simulink model "gm_ZynqBF_2tx_fpga"  (R2018b)
settings: Solver=FixedStepDiscrete  StartTime=0.0  StopTime=10.0  FixedStep=(1/420e3)/128  RelTol=1e-3
undefined symbols (not defined in the file or in its folder): a, b, c
libraries: hdlsllib x873, simulink x349
(part 28 of 40)

== system gm_ZynqBF_2tx_fpga/channel_estimator/peakdetect_ch2/correlator2/correlator_q_instance59 ==
  rx : Inport  OutDataTypeStr=fixdt(1, 16, 15)  PortDimensions=1  SampleTime=1.86011904761905e-08
  gs : Inport  Port=2  OutDataTypeStr=fixdt(1, 16, 15)  PortDimensions=1  SampleTime=1.86011904761905e-08
  start : Inport  Port=3  OutDataTypeStr=boolean  PortDimensions=1  SampleTime=1.86011904761905e-08
  vin : Inport  Port=4  OutDataTypeStr=boolean  PortDimensions=1  SampleTime=1.86011904761905e-08
  Compare To Constant1 : simulink/Logic and Bit Operations/Compare To Constant  relop===  const=fi(0,0,7,0,'hex','3f')  OutDataTypeStr=boolean
  Constant : Constant  Value=0  OutDataTypeStr=fixdt(1, 32, 16)  SampleTime=-1
  Constant1 : Constant  Value=0  OutDataTypeStr=fixdt(1, 16, 15)  SampleTime=-1
  Delay1 : Delay  DelayLength=double(1)  InitialCondition=0  InputProcessing=Inherited  SampleTime=1.86011904761905e-08
  HDL Counter : hdlsllib/Sources/HDL Counter  CountType=Free running  CountInit=double(0)  CountStep=double(1)  CountMax=25  CountFromType=Initial value  CountFrom=double(0)  CountResetPort=on  CountLoadPort=off  CountEnbPort=on  CountDirPort=off  CountDataType=Unsigned  CountWordLen=7  CountFracLen=0  CountSampTime=1.86011904761905e-08
      settings: SourceProductBaseCode=HD
  Multiply-Add : hdlsllib/HDL Operations/Multiply-Add  Function=c+(a.*b)  datatype=fixdt(1, 32, 16)  DoSatur=off  FMA=off
      settings: SourceProductName=HDL Coder  SourceProductBaseCode=HD
  Switch : Switch  Criteria=u2 ~= 0  Threshold=double(0)  OutDataTypeStr=fixdt(1, 32, 16)  SampleTime=1.86011904761905e-08
  Switch1 : Switch  Criteria=u2 ~= 0  Threshold=double(0)  OutDataTypeStr=fixdt(1, 16, 15)  SampleTime=1.86011904761905e-08
  Switch2 : Switch  Criteria=u2 ~= 0  Threshold=double(0)  OutDataTypeStr=fixdt(1, 16, 15)  SampleTime=1.86011904761905e-08
  dout : Outport
  vout : Outport  Port=2
  wires:
  Switch/1 -> Multiply-Add/3
  Delay1/1 -> Switch/3
  vin/1 -> HDL Counter/2, Switch2/2, Switch1/2
  start/1 -> Switch/2, HDL Counter/1
  gs/1 -> Switch2/1
  rx/1 -> Switch1/1
  Compare To Constant1/1 -> vout/1
  Constant/1 -> Switch/1
  Constant1/1 -> Switch2/3, Switch1/3
  HDL Counter/1 -> Compare To Constant1/1
  Multiply-Add/1 -> Delay1/1, dout/1
  Switch1/1 -> Multiply-Add/1
  Switch2/1 -> Multiply-Add/2

== system gm_ZynqBF_2tx_fpga/channel_estimator/peakdetect_ch2/correlator2/correlator_q_instance6 ==
  rx : Inport  OutDataTypeStr=fixdt(1, 16, 15)  PortDimensions=1  SampleTime=1.86011904761905e-08
  gs : Inport  Port=2  OutDataTypeStr=fixdt(1, 16, 15)  PortDimensions=1  SampleTime=1.86011904761905e-08
  start : Inport  Port=3  OutDataTypeStr=boolean  PortDimensions=1  SampleTime=1.86011904761905e-08
  vin : Inport  Port=4  OutDataTypeStr=boolean  PortDimensions=1  SampleTime=1.86011904761905e-08
  Compare To Constant1 : simulink/Logic and Bit Operations/Compare To Constant  relop===  const=fi(0,0,7,0,'hex','3f')  OutDataTypeStr=boolean
  Constant : Constant  Value=0  OutDataTypeStr=fixdt(1, 32, 16)  SampleTime=-1
  Constant1 : Constant  Value=0  OutDataTypeStr=fixdt(1, 16, 15)  SampleTime=-1
  Delay1 : Delay  DelayLength=double(1)  InitialCondition=0  InputProcessing=Inherited  SampleTime=1.86011904761905e-08
  HDL Counter : hdlsllib/Sources/HDL Counter  CountType=Free running  CountInit=double(0)  CountStep=double(1)  CountMax=25  CountFromType=Initial value  CountFrom=double(0)  CountResetPort=on  CountLoadPort=off  CountEnbPort=on  CountDirPort=off  CountDataType=Unsigned  CountWordLen=7  CountFracLen=0  CountSampTime=1.86011904761905e-08
      settings: SourceProductBaseCode=HD
  Multiply-Add : hdlsllib/HDL Operations/Multiply-Add  Function=c+(a.*b)  datatype=fixdt(1, 32, 16)  DoSatur=off  FMA=off
      settings: SourceProductName=HDL Coder  SourceProductBaseCode=HD
  Switch : Switch  Criteria=u2 ~= 0  Threshold=double(0)  OutDataTypeStr=fixdt(1, 32, 16)  SampleTime=1.86011904761905e-08
  Switch1 : Switch  Criteria=u2 ~= 0  Threshold=double(0)  OutDataTypeStr=fixdt(1, 16, 15)  SampleTime=1.86011904761905e-08
  Switch2 : Switch  Criteria=u2 ~= 0  Threshold=double(0)  OutDataTypeStr=fixdt(1, 16, 15)  SampleTime=1.86011904761905e-08
  dout : Outport
  vout : Outport  Port=2
  wires:
  Switch/1 -> Multiply-Add/3
  Delay1/1 -> Switch/3
  vin/1 -> HDL Counter/2, Switch2/2, Switch1/2
  start/1 -> Switch/2, HDL Counter/1
  gs/1 -> Switch2/1
  rx/1 -> Switch1/1
  Compare To Constant1/1 -> vout/1
  Constant/1 -> Switch/1
  Constant1/1 -> Switch2/3, Switch1/3
  HDL Counter/1 -> Compare To Constant1/1
  Multiply-Add/1 -> Delay1/1, dout/1
  Switch1/1 -> Multiply-Add/1
  Switch2/1 -> Multiply-Add/2

== system gm_ZynqBF_2tx_fpga/channel_estimator/peakdetect_ch2/correlator2/correlator_q_instance60 ==
  rx : Inport  OutDataTypeStr=fixdt(1, 16, 15)  PortDimensions=1  SampleTime=1.86011904761905e-08
  gs : Inport  Port=2  OutDataTypeStr=fixdt(1, 16, 15)  PortDimensions=1  SampleTime=1.86011904761905e-08
  start : Inport  Port=3  OutDataTypeStr=boolean  PortDimensions=1  SampleTime=1.86011904761905e-08
  vin : Inport  Port=4  OutDataTypeStr=boolean  PortDimensions=1  SampleTime=1.86011904761905e-08
  Compare To Constant1 : simulink/Logic and Bit Operations/Compare To Constant  relop===  const=fi(0,0,7,0,'hex','3f')  OutDataTypeStr=boolean
  Constant : Constant  Value=0  OutDataTypeStr=fixdt(1, 32, 16)  SampleTime=-1
  Constant1 : Constant  Value=0  OutDataTypeStr=fixdt(1, 16, 15)  SampleTime=-1
  Delay1 : Delay  DelayLength=double(1)  InitialCondition=0  InputProcessing=Inherited  SampleTime=1.86011904761905e-08
  HDL Counter : hdlsllib/Sources/HDL Counter  CountType=Free running  CountInit=double(0)  CountStep=double(1)  CountMax=25  CountFromType=Initial value  CountFrom=double(0)  CountResetPort=on  CountLoadPort=off  CountEnbPort=on  CountDirPort=off  CountDataType=Unsigned  CountWordLen=7  CountFracLen=0  CountSampTime=1.86011904761905e-08
      settings: SourceProductBaseCode=HD
  Multiply-Add : hdlsllib/HDL Operations/Multiply-Add  Function=c+(a.*b)  datatype=fixdt(1, 32, 16)  DoSatur=off  FMA=off
      settings: SourceProductName=HDL Coder  SourceProductBaseCode=HD
  Switch : Switch  Criteria=u2 ~= 0  Threshold=double(0)  OutDataTypeStr=fixdt(1, 32, 16)  SampleTime=1.86011904761905e-08
  Switch1 : Switch  Criteria=u2 ~= 0  Threshold=double(0)  OutDataTypeStr=fixdt(1, 16, 15)  SampleTime=1.86011904761905e-08
  Switch2 : Switch  Criteria=u2 ~= 0  Threshold=double(0)  OutDataTypeStr=fixdt(1, 16, 15)  SampleTime=1.86011904761905e-08
  dout : Outport
  vout : Outport  Port=2
  wires:
  Switch/1 -> Multiply-Add/3
  Delay1/1 -> Switch/3
  vin/1 -> HDL Counter/2, Switch2/2, Switch1/2
  start/1 -> Switch/2, HDL Counter/1
  gs/1 -> Switch2/1
  rx/1 -> Switch1/1
  Compare To Constant1/1 -> vout/1
  Constant/1 -> Switch/1
  Constant1/1 -> Switch2/3, Switch1/3
  HDL Counter/1 -> Compare To Constant1/1
  Multiply-Add/1 -> Delay1/1, dout/1
  Switch1/1 -> Multiply-Add/1
  Switch2/1 -> Multiply-Add/2

== system gm_ZynqBF_2tx_fpga/channel_estimator/peakdetect_ch2/correlator2/correlator_q_instance61 ==
  rx : Inport  OutDataTypeStr=fixdt(1, 16, 15)  PortDimensions=1  SampleTime=1.86011904761905e-08
  gs : Inport  Port=2  OutDataTypeStr=fixdt(1, 16, 15)  PortDimensions=1  SampleTime=1.86011904761905e-08
  start : Inport  Port=3  OutDataTypeStr=boolean  PortDimensions=1  SampleTime=1.86011904761905e-08
  vin : Inport  Port=4  OutDataTypeStr=boolean  PortDimensions=1  SampleTime=1.86011904761905e-08
  Compare To Constant1 : simulink/Logic and Bit Operations/Compare To Constant  relop===  const=fi(0,0,7,0,'hex','3f')  OutDataTypeStr=boolean
  Constant : Constant  Value=0  OutDataTypeStr=fixdt(1, 32, 16)  SampleTime=-1
  Constant1 : Constant  Value=0  OutDataTypeStr=fixdt(1, 16, 15)  SampleTime=-1
  Delay1 : Delay  DelayLength=double(1)  InitialCondition=0  InputProcessing=Inherited  SampleTime=1.86011904761905e-08
  HDL Counter : hdlsllib/Sources/HDL Counter  CountType=Free running  CountInit=double(0)  CountStep=double(1)  CountMax=25  CountFromType=Initial value  CountFrom=double(0)  CountResetPort=on  CountLoadPort=off  CountEnbPort=on  CountDirPort=off  CountDataType=Unsigned  CountWordLen=7  CountFracLen=0  CountSampTime=1.86011904761905e-08
      settings: SourceProductBaseCode=HD
  Multiply-Add : hdlsllib/HDL Operations/Multiply-Add  Function=c+(a.*b)  datatype=fixdt(1, 32, 16)  DoSatur=off  FMA=off
      settings: SourceProductName=HDL Coder  SourceProductBaseCode=HD
  Switch : Switch  Criteria=u2 ~= 0  Threshold=double(0)  OutDataTypeStr=fixdt(1, 32, 16)  SampleTime=1.86011904761905e-08
  Switch1 : Switch  Criteria=u2 ~= 0  Threshold=double(0)  OutDataTypeStr=fixdt(1, 16, 15)  SampleTime=1.86011904761905e-08
  Switch2 : Switch  Criteria=u2 ~= 0  Threshold=double(0)  OutDataTypeStr=fixdt(1, 16, 15)  SampleTime=1.86011904761905e-08
  dout : Outport
  vout : Outport  Port=2
  wires:
  Switch/1 -> Multiply-Add/3
  Delay1/1 -> Switch/3
  vin/1 -> HDL Counter/2, Switch2/2, Switch1/2
  start/1 -> Switch/2, HDL Counter/1
  gs/1 -> Switch2/1
  rx/1 -> Switch1/1
  Compare To Constant1/1 -> vout/1
  Constant/1 -> Switch/1
  Constant1/1 -> Switch2/3, Switch1/3
  HDL Counter/1 -> Compare To Constant1/1
  Multiply-Add/1 -> Delay1/1, dout/1
  Switch1/1 -> Multiply-Add/1
  Switch2/1 -> Multiply-Add/2

== system gm_ZynqBF_2tx_fpga/channel_estimator/peakdetect_ch2/correlator2/correlator_q_instance62 ==
  rx : Inport  OutDataTypeStr=fixdt(1, 16, 15)  PortDimensions=1  SampleTime=1.86011904761905e-08
  gs : Inport  Port=2  OutDataTypeStr=fixdt(1, 16, 15)  PortDimensions=1  SampleTime=1.86011904761905e-08
  start : Inport  Port=3  OutDataTypeStr=boolean  PortDimensions=1  SampleTime=1.86011904761905e-08
  vin : Inport  Port=4  OutDataTypeStr=boolean  PortDimensions=1  SampleTime=1.86011904761905e-08
  Compare To Constant1 : simulink/Logic and Bit Operations/Compare To Constant  relop===  const=fi(0,0,7,0,'hex','3f')  OutDataTypeStr=boolean
  Constant : Constant  Value=0  OutDataTypeStr=fixdt(1, 32, 16)  SampleTime=-1
  Constant1 : Constant  Value=0  OutDataTypeStr=fixdt(1, 16, 15)  SampleTime=-1
  Delay1 : Delay  DelayLength=double(1)  InitialCondition=0  InputProcessing=Inherited  SampleTime=1.86011904761905e-08
  HDL Counter : hdlsllib/Sources/HDL Counter  CountType=Free running  CountInit=double(0)  CountStep=double(1)  CountMax=25  CountFromType=Initial value  CountFrom=double(0)  CountResetPort=on  CountLoadPort=off  CountEnbPort=on  CountDirPort=off  CountDataType=Unsigned  CountWordLen=7  CountFracLen=0  CountSampTime=1.86011904761905e-08
      settings: SourceProductBaseCode=HD
  Multiply-Add : hdlsllib/HDL Operations/Multiply-Add  Function=c+(a.*b)  datatype=fixdt(1, 32, 16)  DoSatur=off  FMA=off
      settings: SourceProductName=HDL Coder  SourceProductBaseCode=HD
  Switch : Switch  Criteria=u2 ~= 0  Threshold=double(0)  OutDataTypeStr=fixdt(1, 32, 16)  SampleTime=1.86011904761905e-08
  Switch1 : Switch  Criteria=u2 ~= 0  Threshold=double(0)  OutDataTypeStr=fixdt(1, 16, 15)  SampleTime=1.86011904761905e-08
  Switch2 : Switch  Criteria=u2 ~= 0  Threshold=double(0)  OutDataTypeStr=fixdt(1, 16, 15)  SampleTime=1.86011904761905e-08
  dout : Outport
  vout : Outport  Port=2
  wires:
  Switch/1 -> Multiply-Add/3
  Delay1/1 -> Switch/3
  vin/1 -> HDL Counter/2, Switch2/2, Switch1/2
  start/1 -> Switch/2, HDL Counter/1
  gs/1 -> Switch2/1
  rx/1 -> Switch1/1
  Compare To Constant1/1 -> vout/1
  Constant/1 -> Switch/1
  Constant1/1 -> Switch2/3, Switch1/3
  HDL Counter/1 -> Compare To Constant1/1
  Multiply-Add/1 -> Delay1/1, dout/1
  Switch1/1 -> Multiply-Add/1
  Switch2/1 -> Multiply-Add/2

== system gm_ZynqBF_2tx_fpga/channel_estimator/peakdetect_ch2/correlator2/correlator_q_instance63 ==
  rx : Inport  OutDataTypeStr=fixdt(1, 16, 15)  PortDimensions=1  SampleTime=1.86011904761905e-08
  gs : Inport  Port=2  OutDataTypeStr=fixdt(1, 16, 15)  PortDimensions=1  SampleTime=1.86011904761905e-08
  start : Inport  Port=3  OutDataTypeStr=boolean  PortDimensions=1  SampleTime=1.86011904761905e-08
  vin : Inport  Port=4  OutDataTypeStr=boolean  PortDimensions=1  SampleTime=1.86011904761905e-08
  Compare To Constant1 : simulink/Logic and Bit Operations/Compare To Constant  relop===  const=fi(0,0,7,0,'hex','3f')  OutDataTypeStr=boolean
  Constant : Constant  Value=0  OutDataTypeStr=fixdt(1, 32, 16)  SampleTime=-1
  Constant1 : Constant  Value=0  OutDataTypeStr=fixdt(1, 16, 15)  SampleTime=-1
  Delay1 : Delay  DelayLength=double(1)  InitialCondition=0  InputProcessing=Inherited  SampleTime=1.86011904761905e-08
  HDL Counter : hdlsllib/Sources/HDL Counter  CountType=Free running  CountInit=double(0)  CountStep=double(1)  CountMax=25  CountFromType=Initial value  CountFrom=double(0)  CountResetPort=on  CountLoadPort=off  CountEnbPort=on  CountDirPort=off  CountDataType=Unsigned  CountWordLen=7  CountFracLen=0  CountSampTime=1.86011904761905e-08
      settings: SourceProductBaseCode=HD
  Multiply-Add : hdlsllib/HDL Operations/Multiply-Add  Function=c+(a.*b)  datatype=fixdt(1, 32, 16)  DoSatur=off  FMA=off
      settings: SourceProductName=HDL Coder  SourceProductBaseCode=HD
  Switch : Switch  Criteria=u2 ~= 0  Threshold=double(0)  OutDataTypeStr=fixdt(1, 32, 16)  SampleTime=1.86011904761905e-08
  Switch1 : Switch  Criteria=u2 ~= 0  Threshold=double(0)  OutDataTypeStr=fixdt(1, 16, 15)  SampleTime=1.86011904761905e-08
  Switch2 : Switch  Criteria=u2 ~= 0  Threshold=double(0)  OutDataTypeStr=fixdt(1, 16, 15)  SampleTime=1.86011904761905e-08
  dout : Outport
  vout : Outport  Port=2
  wires:
  Switch/1 -> Multiply-Add/3
  Delay1/1 -> Switch/3
  vin/1 -> HDL Counter/2, Switch2/2, Switch1/2
  start/1 -> Switch/2, HDL Counter/1
  gs/1 -> Switch2/1
  rx/1 -> Switch1/1
  Compare To Constant1/1 -> vout/1
  Constant/1 -> Switch/1
  Constant1/1 -> Switch2/3, Switch1/3
  HDL Counter/1 -> Compare To Constant1/1
  Multiply-Add/1 -> Delay1/1, dout/1
  Switch1/1 -> Multiply-Add/1
  Switch2/1 -> Multiply-Add/2

== system gm_ZynqBF_2tx_fpga/channel_estimator/peakdetect_ch2/correlator2/correlator_q_instance64 ==
  rx : Inport  OutDataTypeStr=fixdt(1, 16, 15)  PortDimensions=1  SampleTime=1.86011904761905e-08
  gs : Inport  Port=2  OutDataTypeStr=fixdt(1, 16, 15)  PortDimensions=1  SampleTime=1.86011904761905e-08
  start : Inport  Port=3  OutDataTypeStr=boolean  PortDimensions=1  SampleTime=1.86011904761905e-08
  vin : Inport  Port=4  OutDataTypeStr=boolean  PortDimensions=1  SampleTime=1.86011904761905e-08
  Compare To Constant1 : simulink/Logic and Bit Operations/Compare To Constant  relop===  const=fi(0,0,7,0,'hex','3f')  OutDataTypeStr=boolean
  Constant : Constant  Value=0  OutDataTypeStr=fixdt(1, 32, 16)  SampleTime=-1
  Constant1 : Constant  Value=0  OutDataTypeStr=fixdt(1, 16, 15)  SampleTime=-1
  Delay1 : Delay  DelayLength=double(1)  InitialCondition=0  InputProcessing=Inherited  SampleTime=1.86011904761905e-08
  HDL Counter : hdlsllib/Sources/HDL Counter  CountType=Free running  CountInit=double(0)  CountStep=double(1)  CountMax=25  CountFromType=Initial value  CountFrom=double(0)  CountResetPort=on  CountLoadPort=off  CountEnbPort=on  CountDirPort=off  CountDataType=Unsigned  CountWordLen=7  CountFracLen=0  CountSampTime=1.86011904761905e-08
      settings: SourceProductBaseCode=HD
  Multiply-Add : hdlsllib/HDL Operations/Multiply-Add  Function=c+(a.*b)  datatype=fixdt(1, 32, 16)  DoSatur=off  FMA=off
      settings: SourceProductName=HDL Coder  SourceProductBaseCode=HD
  Switch : Switch  Criteria=u2 ~= 0  Threshold=double(0)  OutDataTypeStr=fixdt(1, 32, 16)  SampleTime=1.86011904761905e-08
  Switch1 : Switch  Criteria=u2 ~= 0  Threshold=double(0)  OutDataTypeStr=fixdt(1, 16, 15)  SampleTime=1.86011904761905e-08
  Switch2 : Switch  Criteria=u2 ~= 0  Threshold=double(0)  OutDataTypeStr=fixdt(1, 16, 15)  SampleTime=1.86011904761905e-08
  dout : Outport
  vout : Outport  Port=2
  wires:
  Switch/1 -> Multiply-Add/3
  Delay1/1 -> Switch/3
  vin/1 -> HDL Counter/2, Switch2/2, Switch1/2
  start/1 -> Switch/2, HDL Counter/1
  gs/1 -> Switch2/1
  rx/1 -> Switch1/1
  Compare To Constant1/1 -> vout/1
  Constant/1 -> Switch/1
  Constant1/1 -> Switch2/3, Switch1/3
  HDL Counter/1 -> Compare To Constant1/1
  Multiply-Add/1 -> Delay1/1, dout/1
  Switch1/1 -> Multiply-Add/1
  Switch2/1 -> Multiply-Add/2

== system gm_ZynqBF_2tx_fpga/channel_estimator/peakdetect_ch2/correlator2/correlator_q_instance7 ==
  rx : Inport  OutDataTypeStr=fixdt(1, 16, 15)  PortDimensions=1  SampleTime=1.86011904761905e-08
  gs : Inport  Port=2  OutDataTypeStr=fixdt(1, 16, 15)  PortDimensions=1  SampleTime=1.86011904761905e-08
  start : Inport  Port=3  OutDataTypeStr=boolean  PortDimensions=1  SampleTime=1.86011904761905e-08
  vin : Inport  Port=4  OutDataTypeStr=boolean  PortDimensions=1  SampleTime=1.86011904761905e-08
  Compare To Constant1 : simulink/Logic and Bit Operations/Compare To Constant  relop===  const=fi(0,0,7,0,'hex','3f')  OutDataTypeStr=boolean
  Constant : Constant  Value=0  OutDataTypeStr=fixdt(1, 32, 16)  SampleTime=-1
  Constant1 : Constant  Value=0  OutDataTypeStr=fixdt(1, 16, 15)  SampleTime=-1
  Delay1 : Delay  DelayLength=double(1)  InitialCondition=0  InputProcessing=Inherited  SampleTime=1.86011904761905e-08
  HDL Counter : hdlsllib/Sources/HDL Counter  CountType=Free running  CountInit=double(0)  CountStep=double(1)  CountMax=25  CountFromType=Initial value  CountFrom=double(0)  CountResetPort=on  CountLoadPort=off  CountEnbPort=on  CountDirPort=off  CountDataType=Unsigned  CountWordLen=7  CountFracLen=0  CountSampTime=1.86011904761905e-08
      settings: SourceProductBaseCode=HD
  Multiply-Add : hdlsllib/HDL Operations/Multiply-Add  Function=c+(a.*b)  datatype=fixdt(1, 32, 16)  DoSatur=off  FMA=off
      settings: SourceProductName=HDL Coder  SourceProductBaseCode=HD
  Switch : Switch  Criteria=u2 ~= 0  Threshold=double(0)  OutDataTypeStr=fixdt(1, 32, 16)  SampleTime=1.86011904761905e-08
  Switch1 : Switch  Criteria=u2 ~= 0  Threshold=double(0)  OutDataTypeStr=fixdt(1, 16, 15)  SampleTime=1.86011904761905e-08
  Switch2 : Switch  Criteria=u2 ~= 0  Threshold=double(0)  OutDataTypeStr=fixdt(1, 16, 15)  SampleTime=1.86011904761905e-08
  dout : Outport
  vout : Outport  Port=2
  wires:
  Switch/1 -> Multiply-Add/3
  Delay1/1 -> Switch/3
  vin/1 -> HDL Counter/2, Switch2/2, Switch1/2
  start/1 -> Switch/2, HDL Counter/1
  gs/1 -> Switch2/1
  rx/1 -> Switch1/1
  Compare To Constant1/1 -> vout/1
  Constant/1 -> Switch/1
  Constant1/1 -> Switch2/3, Switch1/3
  HDL Counter/1 -> Compare To Constant1/1
  Multiply-Add/1 -> Delay1/1, dout/1
  Switch1/1 -> Multiply-Add/1
  Switch2/1 -> Multiply-Add/2

== system gm_ZynqBF_2tx_fpga/channel_estimator/peakdetect_ch2/correlator2/correlator_q_instance8 ==
  rx : Inport  OutDataTypeStr=fixdt(1, 16, 15)  PortDimensions=1  SampleTime=1.86011904761905e-08
  gs : Inport  Port=2  OutDataTypeStr=fixdt(1, 16, 15)  PortDimensions=1  SampleTime=1.86011904761905e-08
  start : Inport  Port=3  OutDataTypeStr=boolean  PortDimensions=1  SampleTime=1.86011904761905e-08
  vin : Inport  Port=4  OutDataTypeStr=boolean  PortDimensions=1  SampleTime=1.86011904761905e-08
  Compare To Constant1 : simulink/Logic and Bit Operations/Compare To Constant  relop===  const=fi(0,0,7,0,'hex','3f')  OutDataTypeStr=boolean
  Constant : Constant  Value=0  OutDataTypeStr=fixdt(1, 32, 16)  SampleTime=-1
  Constant1 : Constant  Value=0  OutDataTypeStr=fixdt(1, 16, 15)  SampleTime=-1
  Delay1 : Delay  DelayLength=double(1)  InitialCondition=0  InputProcessing=Inherited  SampleTime=1.86011904761905e-08
  HDL Counter : hdlsllib/Sources/HDL Counter  CountType=Free running  CountInit=double(0)  CountStep=double(1)  CountMax=25  CountFromType=Initial value  CountFrom=double(0)  CountResetPort=on  CountLoadPort=off  CountEnbPort=on  CountDirPort=off  CountDataType=Unsigned  CountWordLen=7  CountFracLen=0  CountSampTime=1.86011904761905e-08
      settings: SourceProductBaseCode=HD
  Multiply-Add : hdlsllib/HDL Operations/Multiply-Add  Function=c+(a.*b)  datatype=fixdt(1, 32, 16)  DoSatur=off  FMA=off
      settings: SourceProductName=HDL Coder  SourceProductBaseCode=HD
  Switch : Switch  Criteria=u2 ~= 0  Threshold=double(0)  OutDataTypeStr=fixdt(1, 32, 16)  SampleTime=1.86011904761905e-08
  Switch1 : Switch  Criteria=u2 ~= 0  Threshold=double(0)  OutDataTypeStr=fixdt(1, 16, 15)  SampleTime=1.86011904761905e-08
  Switch2 : Switch  Criteria=u2 ~= 0  Threshold=double(0)  OutDataTypeStr=fixdt(1, 16, 15)  SampleTime=1.86011904761905e-08
  dout : Outport
  vout : Outport  Port=2
  wires:
  Switch/1 -> Multiply-Add/3
  Delay1/1 -> Switch/3
  vin/1 -> HDL Counter/2, Switch2/2, Switch1/2
  start/1 -> Switch/2, HDL Counter/1
  gs/1 -> Switch2/1
  rx/1 -> Switch1/1
  Compare To Constant1/1 -> vout/1
  Constant/1 -> Switch/1
  Constant1/1 -> Switch2/3, Switch1/3
  HDL Counter/1 -> Compare To Constant1/1
  Multiply-Add/1 -> Delay1/1, dout/1
  Switch1/1 -> Multiply-Add/1
  Switch2/1 -> Multiply-Add/2

== system gm_ZynqBF_2tx_fpga/channel_estimator/peakdetect_ch2/correlator2/correlator_q_instance9 ==
  rx : Inport  OutDataTypeStr=fixdt(1, 16, 15)  PortDimensions=1  SampleTime=1.86011904761905e-08
  gs : Inport  Port=2  OutDataTypeStr=fixdt(1, 16, 15)  PortDimensions=1  SampleTime=1.86011904761905e-08
  start : Inport  Port=3  OutDataTypeStr=boolean  PortDimensions=1  SampleTime=1.86011904761905e-08
  vin : Inport  Port=4  OutDataTypeStr=boolean  PortDimensions=1  SampleTime=1.86011904761905e-08
  Compare To Constant1 : simulink/Logic and Bit Operations/Compare To Constant  relop===  const=fi(0,0,7,0,'hex','3f')  OutDataTypeStr=boolean
  Constant : Constant  Value=0  OutDataTypeStr=fixdt(1, 32, 16)  SampleTime=-1
  Constant1 : Constant  Value=0  OutDataTypeStr=fixdt(1, 16, 15)  SampleTime=-1
  Delay1 : Delay  DelayLength=double(1)  InitialCondition=0  InputProcessing=Inherited  SampleTime=1.86011904761905e-08
  HDL Counter : hdlsllib/Sources/HDL Counter  CountType=Free running  CountInit=double(0)  CountStep=double(1)  CountMax=25  CountFromType=Initial value  CountFrom=double(0)  CountResetPort=on  CountLoadPort=off  CountEnbPort=on  CountDirPort=off  CountDataType=Unsigned  CountWordLen=7  CountFracLen=0  CountSampTime=1.86011904761905e-08
      settings: SourceProductBaseCode=HD
  Multiply-Add : hdlsllib/HDL Operations/Multiply-Add  Function=c+(a.*b)  datatype=fixdt(1, 32, 16)  DoSatur=off  FMA=off
      settings: SourceProductName=HDL Coder  SourceProductBaseCode=HD
  Switch : Switch  Criteria=u2 ~= 0  Threshold=double(0)  OutDataTypeStr=fixdt(1, 32, 16)  SampleTime=1.86011904761905e-08
  Switch1 : Switch  Criteria=u2 ~= 0  Threshold=double(0)  OutDataTypeStr=fixdt(1, 16, 15)  SampleTime=1.86011904761905e-08
  Switch2 : Switch  Criteria=u2 ~= 0  Threshold=double(0)  OutDataTypeStr=fixdt(1, 16, 15)  SampleTime=1.86011904761905e-08
  dout : Outport
  vout : Outport  Port=2
  wires:
  Switch/1 -> Multiply-Add/3
  Delay1/1 -> Switch/3
  vin/1 -> HDL Counter/2, Switch2/2, Switch1/2
  start/1 -> Switch/2, HDL Counter/1
  gs/1 -> Switch2/1
  rx/1 -> Switch1/1
  Compare To Constant1/1 -> vout/1
  Constant/1 -> Switch/1
  Constant1/1 -> Switch2/3, Switch1/3
  HDL Counter/1 -> Compare To Constant1/1
  Multiply-Add/1 -> Delay1/1, dout/1
  Switch1/1 -> Multiply-Add/1
  Switch2/1 -> Multiply-Add/2

== system gm_ZynqBF_2tx_fpga/channel_estimator/peakdetect_ch2/correlator2/data_in ==
  rst : Inport  OutDataTypeStr=boolean  PortDimensions=1  SampleTime=1.86011904761905e-08
  valid : Inport  Port=2  OutDataTypeStr=boolean  PortDimensions=1  SampleTime=1.86011904761905e-08
  Bit Rotate : hdlsllib/Logic and Bit Operations/Bit Rotate  mode=Rotate Left  N=double(1)
      settings: SourceProductName=HDL Coder  SourceProductBaseCode=HD
  Compare To Constant : simulink/Logic and Bit Operations/Compare To Constant  relop===  const=fi(0,0,6,0,'hex','3f')  OutDataTypeStr=boolean
  Constant1 : Constant  Value=0  OutDataTypeStr=fixdt(0, 64, 0)  SampleTime=-1
  Delay{,1..4,6} (6 alike) : Delay  DelayLength=double(1)  InitialCondition=0  InputProcessing=Inherited  SampleTime=1.86011904761905e-08
  Delay1_Initial_Val : Constant  Value=9223372036854775808  OutDataTypeStr=fixdt(0, 64, 0)  SampleTime=-1
  Delay1_ctrl_const : Constant  OutDataTypeStr=boolean  SampleTime=1.86011904761905e-08
  Delay1_ctrl_delay : Delay  DelayLength=double(1)  InitialCondition=0  InputProcessing=Inherited  SampleTime=1.86011904761905e-08
  Delay1_switch : Switch  Criteria=u2 ~= 0  Threshold=double(0)  OutDataTypeStr=fixdt(0, 64, 0)  SampleTime=1.86011904761905e-08
  Delay5 : Delay  DelayLength=double(3)  InitialCondition=0  InputProcessing=Inherited  SampleTime=1.86011904761905e-08
  Logical Operator : Logic  AllPortsSameDT=off  OutDataTypeStr=boolean  SampleTime=1.86011904761905e-08
  Switch1 : Switch  Criteria=u2 ~= 0  Threshold=double(0)  OutDataTypeStr=fixdt(0, 64, 0)  SampleTime=1.86011904761905e-08
  Switch2 : Switch  Criteria=u2 ~= 0  Threshold=double(0)  OutDataTypeStr=fixdt(0, 64, 0)  SampleTime=1.86011904761905e-08
  addr_counter : hdlsllib/Sources/HDL Counter  CountType=Count limited  CountInit=double(63)  CountStep=double(1)  CountMax=double(511)  CountFromType=Initial value  CountFrom=double(63)  CountResetPort=on  CountLoadPort=off  CountEnbPort=on  CountDirPort=off  CountDataType=Unsigned  CountWordLen=9  CountFracLen=0  CountSampTime=1.86011904761905e-08
      settings: SourceProductBaseCode=HD
  ram_counter : hdlsllib/Sources/HDL Counter  CountType=Free running  CountInit=double(63)  CountStep=double(1)  CountMax=25  CountFromType=Initial value  CountFrom=double(63)  CountResetPort=on  CountLoadPort=off  CountEnbPort=on  CountDirPort=off  CountDataType=Unsigned  CountWordLen=6  CountFracLen=0  CountSampTime=1.86011904761905e-08
      settings: SourceProductBaseCode=HD
  addr : Outport
  we : Outport  Port=2
  wires:
  rst/1 -> Delay4/1
  valid/1 -> Delay3/1
  Bit Rotate/1 -> Switch1/1
  Compare To Constant/1 -> Logical Operator/1
  Constant1/1 -> Switch2/3
  Delay/1 -> Switch2/2
  Delay1_switch/1 -> Switch1/3, Bit Rotate/1
  Delay2/1 -> we/1
  Delay3/1 -> Logical Operator/2, ram_counter/2, Delay6/1
  Delay4/1 -> ram_counter/1, addr_counter/1
  Delay5/1 -> addr/1
  Delay6/1 -> Switch1/2, Delay/1
  Logical Operator/1 -> addr_counter/2
  Switch1/1 -> Switch2/1, Delay1/1
  Switch2/1 -> Delay2/1
  addr_counter/1 -> Delay5/1
  ram_counter/1 -> Compare To Constant/1
  Delay1/1 -> Delay1_switch/1
  Delay1_Initial_Val/1 -> Delay1_switch/3
  Delay1_ctrl_const/1 -> Delay1_ctrl_delay/1
  Delay1_ctrl_delay/1 -> Delay1_switch/2
